simulink model "Position_Sliding_Mode"  (R2024b)
settings: Solver=ode4  StartTime=0.0  StopTime=20  FixedStep=dT  RelTol=1e-3
InitFcn:
  | O = [0; 0; 0];        % world origin frame
  | C = [0.0; 0.0; 0.0];  % camera origin frame
  | 
  | d_initial = C - O;            % distance between camera and world frame
  | ang_initial = [0.0 0.0 0.0];  % initial orientation, [pi 0 pi/2]
  | ang_final = [0.0*pi/180  0.0*pi/180  0.0*pi/180];
  | init_pose = [C ; ang_initial'];
  | d_final=[0; 0; 3];
  | dT=0.25;
  | g = 9.81;
  | mass = 1; L = 0.2;
  | Ix = 0.008;
  | Iy = 0.015;
  | Iz = 0.017;
  | c = 0.088;
settings Model: Creator=k513  LastModifiedBy=mohsen
settings ModelReferenceCC: EnableRefExpFcnMdlSchedulingChecks=on
settings RTWCC: GPUComputeCapability=3.5

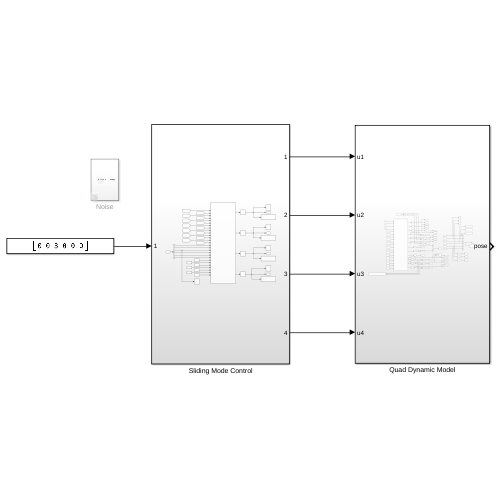
[thumbnail: Simulink's stored preview of the top-level diagram]
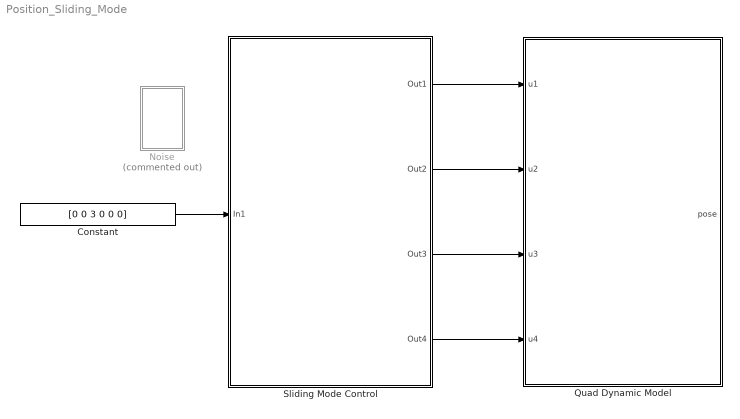
== system Position_Sliding_Mode ==
  Constant : Constant  Value=[0 0 3 0 0 0]
  Noise : Subsystem  Commented=on
  Quad Dynamic Model : Subsystem
  Sliding Mode Control : Subsystem
  wires:
  Sliding Mode Control/1(Out1) -> Quad Dynamic Model/1(u1)
  Sliding Mode Control/3(Out3) -> Quad Dynamic Model/3(u3)
  Sliding Mode Control/2(Out2) -> Quad Dynamic Model/2(u2)
  Sliding Mode Control/4(Out4) -> Quad Dynamic Model/4(u4)
  Constant/1 -> Sliding Mode Control/1(In1)

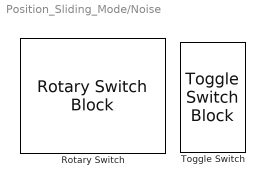
== system Position_Sliding_Mode/Noise ==
  Rotary Switch : RotarySwitchBlock  LabelPosition=Bottom
      settings: Values={{'Off', 'Low', 'Medium', 'High'}, [0 0.1 0.2 0.3]}
  Toggle Switch : ToggleSwitchBlock  LabelPosition=Bottom
      settings: Values={{'Off', 'On'}, [0 1]}

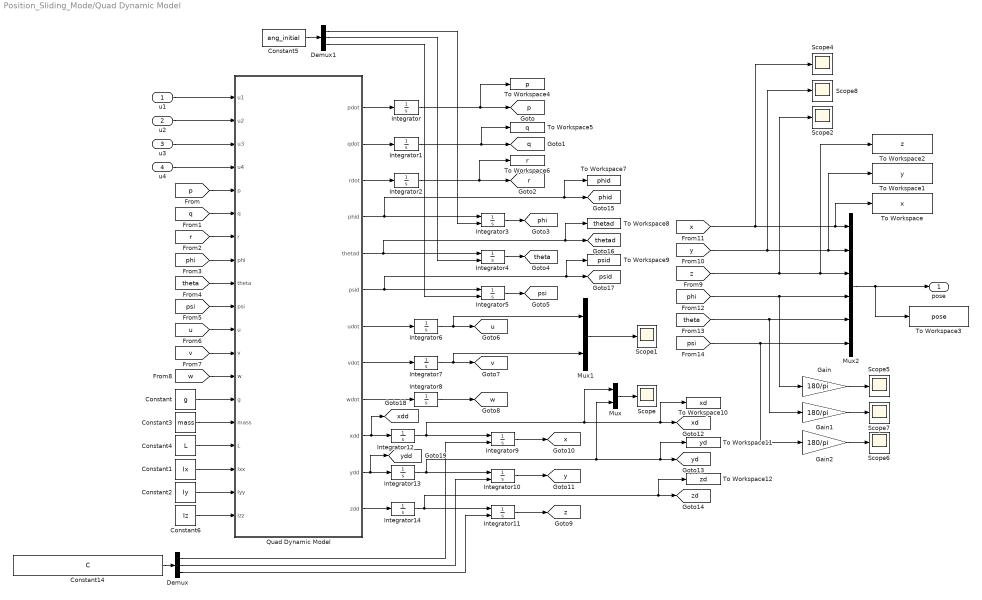
== system Position_Sliding_Mode/Quad Dynamic Model ==
  u1 : Inport
  u2 : Inport  Port=2
  u3 : Inport  Port=3
  u4 : Inport  Port=4
  Constant : Constant  Value=g
  Constant1 : Constant  Value=Ix
  Constant14 : Constant  Value=C
  Constant2 : Constant  Value=Iy
  Constant3 : Constant  Value=mass
  Constant4 : Constant  Value=L
  Constant5 : Constant  Value=ang_initial
  Constant6 : Constant  Value=Iz
  Demux : Demux  Outputs=3
  Demux1 : Demux  Outputs=3
  Gain : Gain  Gain=180/pi
  Gain1 : Gain  Gain=180/pi
  Gain2 : Gain  Gain=180/pi
  Integrator : Integrator  InitialCondition=-0.003775510005653
  Integrator1 : Integrator  InitialCondition=0.003931066952646
  Integrator{3..5,9..11} (6 alike) : Integrator  InitialConditionSource=external
  Integrator{6..8,12..14} (6 alike) : Integrator
  Integrator2 : Integrator  InitialCondition=0.005723309703171
  Mux : Mux  Inputs=2
  Mux1 : Mux  Inputs=2
  Mux2 : Mux  Inputs=6
  Quad Dynamic Model : MATLAB Function  TreatAsAtomicUnit=on
  Scope{,1..2,4..8} (8 alike) : Scope
  To Workspace : ToWorkspace  VariableName=x  SampleTime=-1
      settings: Save2DSignal=2-D array (concatenate along first dimension)
  To Workspace1 : ToWorkspace  VariableName=y  SampleTime=-1
      settings: Save2DSignal=2-D array (concatenate along first dimension)
  To Workspace10 : ToWorkspace  VariableName=xd  SampleTime=-1
  To Workspace11 : ToWorkspace  VariableName=yd  SampleTime=-1
  To Workspace12 : ToWorkspace  VariableName=zd  SampleTime=-1
  To Workspace2 : ToWorkspace  VariableName=z  SampleTime=-1
      settings: Save2DSignal=2-D array (concatenate along first dimension)
  To Workspace3 : ToWorkspace  VariableName=pose  SampleTime=-1
      settings: Save2DSignal=2-D array (concatenate along first dimension)
  To Workspace4 : ToWorkspace  VariableName=p  SampleTime=-1
  To Workspace5 : ToWorkspace  VariableName=q  SampleTime=-1
  To Workspace6 : ToWorkspace  VariableName=r  SampleTime=-1
  To Workspace7 : ToWorkspace  VariableName=phid  SampleTime=-1
  To Workspace8 : ToWorkspace  VariableName=thetad  SampleTime=-1
  To Workspace9 : ToWorkspace  VariableName=psid  SampleTime=-1
  pose : Outport
  tag scope: p=global, phi=global, phid=global, psi=global, psid=global, q=global, r=global, theta=global, thetad=global, u=global, v=global, w=global, x=global, xd=global, xdd=global, y=global, yd=global, ydd=global, z=global, zd=global
  wires:
  Quad Dynamic Model/1(pdot) -> Integrator/1
  Quad Dynamic Model/2(qdot) -> Integrator1/1
  Quad Dynamic Model/3(rdot) -> Integrator2/1
  Quad Dynamic Model/4(phid) -> To Workspace7/1, [phid], Integrator3/1
  Quad Dynamic Model/5(thetad) -> To Workspace8/1, [thetad], Integrator4/1
  Quad Dynamic Model/7(udot) -> Integrator6/1
  Quad Dynamic Model/9(wdot) -> Integrator8/1
  Quad Dynamic Model/10(xdd) -> [xdd], Integrator12/1
  Quad Dynamic Model/11(ydd) -> [ydd], Integrator13/1
  Quad Dynamic Model/12(zdd) -> Integrator14/1
  Integrator1/1 -> To Workspace5/1, [q]
  Integrator2/1 -> To Workspace6/1, [r]
  Integrator3/1 -> [phi]
  Integrator4/1 -> [theta]
  Integrator5/1 -> [psi]
  Integrator6/1 -> [u], Mux1/1
  Integrator7/1 -> [v], Mux1/2
  Integrator8/1 -> [w]
  [p] -> Quad Dynamic Model/5(p)
  [q] -> Quad Dynamic Model/6(q)
  [r] -> Quad Dynamic Model/7(r)
  [phi] -> Quad Dynamic Model/8(phi)
  [theta] -> Quad Dynamic Model/9(theta)
  [psi] -> Quad Dynamic Model/10(psi)
  [u] -> Quad Dynamic Model/11(u)
  [v] -> Quad Dynamic Model/12(v)
  [w] -> Quad Dynamic Model/13(w)
  Integrator9/1 -> [x]
  Integrator10/1 -> [y]
  Integrator11/1 -> [z]
  u1/1 -> Quad Dynamic Model/1(u1)
  u2/1 -> Quad Dynamic Model/2(u2)
  u3/1 -> Quad Dynamic Model/3(u3)
  u4/1 -> Quad Dynamic Model/4(u4)
  Integrator12/1 -> Mux/1, To Workspace10/1, [xd], Integrator9/1
  Integrator13/1 -> Mux/2, To Workspace11/1, [yd], Integrator10/1
  Integrator14/1 -> To Workspace12/1, [zd], Integrator11/1
  Quad Dynamic Model/6(psid) -> Integrator5/1, To Workspace9/1, [psid]
  Demux/1 -> Integrator9/2
  Demux/2 -> Integrator10/2
  Demux/3 -> Integrator11/2
  Mux/1 -> Scope/1
  Mux1/1 -> Scope1/1
  Constant14/1 -> Demux/1
  Quad Dynamic Model/8(vdot) -> Integrator7/1
  [x] -> Mux2/1, To Workspace/1, Scope4/1
  [phi] -> Gain/1, Mux2/4
  [psi] -> Mux2/6, Gain2/1
  [theta] -> Gain1/1, Mux2/5
  Gain/1 -> Scope5/1
  Gain1/1 -> Scope7/1
  Gain2/1 -> Scope6/1
  [y] -> Mux2/2, To Workspace1/1, Scope8/1
  [z] -> To Workspace2/1, Mux2/3, Scope2/1
  Mux2/1 -> pose/1, To Workspace3/1
  Constant/1 -> Quad Dynamic Model/14(g)
  Constant2/1 -> Quad Dynamic Model/18(Iyy)
  Constant1/1 -> Quad Dynamic Model/17(Ixx)
  Constant3/1 -> Quad Dynamic Model/15(mass)
  Constant4/1 -> Quad Dynamic Model/16(L)
  Constant5/1 -> Demux1/1
  Demux1/1 -> Integrator3/2
  Demux1/2 -> Integrator4/2
  Demux1/3 -> Integrator5/2
  Constant6/1 -> Quad Dynamic Model/19(Izz)
  Integrator/1 -> To Workspace4/1, [p]

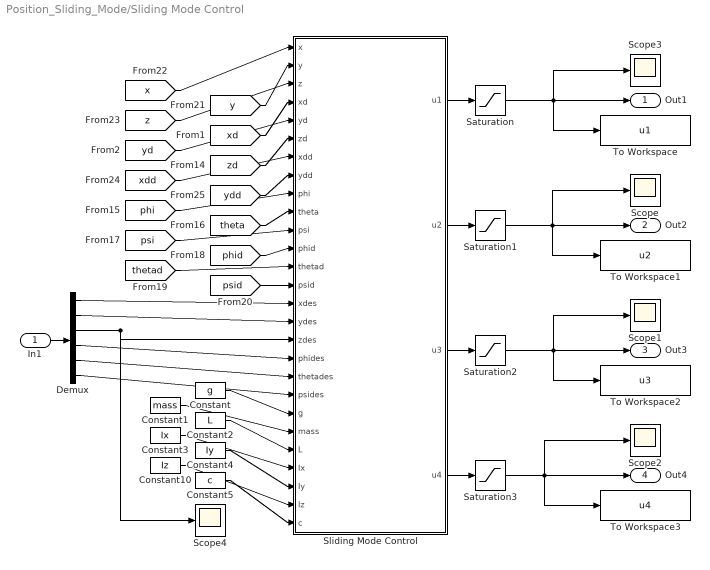
== system Position_Sliding_Mode/Sliding Mode Control ==
  In1 : Inport
  Constant : Constant  Value=g
  Constant1 : Constant  Value=mass
  Constant10 : Constant  Value=Iz
  Constant2 : Constant  Value=L
  Constant3 : Constant  Value=Ix
  Constant4 : Constant  Value=Iy
  Constant5 : Constant  Value=c
  Demux : Demux  Outputs=6
  Saturation : Saturate  UpperLimit=13  LowerLimit=9
  Saturation1 : Saturate  UpperLimit=8  LowerLimit=-8
  Saturation2 : Saturate  UpperLimit=8  LowerLimit=-8
  Saturation3 : Saturate  UpperLimit=4  LowerLimit=-3
  Scope{,1..4} (5 alike) : Scope
  Sliding Mode Control : MATLAB Function  TreatAsAtomicUnit=on
  To Workspace : ToWorkspace  VariableName=u1  SaveFormat=Timeseries  SampleTime=-1
  To Workspace1 : ToWorkspace  VariableName=u2  SaveFormat=Timeseries  SampleTime=-1
  To Workspace2 : ToWorkspace  VariableName=u3  SaveFormat=Timeseries  SampleTime=-1
  To Workspace3 : ToWorkspace  VariableName=u4  SaveFormat=Timeseries  SampleTime=-1
  Out1 : Outport
  Out2 : Outport  Port=2
  Out3 : Outport  Port=3
  Out4 : Outport  Port=4
  wires:
  [theta] -> Sliding Mode Control/10(theta)
  [zd] -> Sliding Mode Control/6(zd)
  [yd] -> Sliding Mode Control/5(yd)
  Sliding Mode Control/1(u1) -> Saturation/1
  [xdd] -> Sliding Mode Control/7(xdd)
  [thetad] -> Sliding Mode Control/13(thetad)
  [phid] -> Sliding Mode Control/12(phid)
  [psi] -> Sliding Mode Control/11(psi)
  Saturation/1 -> To Workspace/1, Out1/1, Scope3/1
  [ydd] -> Sliding Mode Control/8(ydd)
  [y] -> Sliding Mode Control/2(y)
  [phi] -> Sliding Mode Control/9(phi)
  [xd] -> Sliding Mode Control/4(xd)
  Sliding Mode Control/4(u4) -> Saturation3/1
  Sliding Mode Control/2(u2) -> Saturation1/1
  [psid] -> Sliding Mode Control/14(psid)
  [x] -> Sliding Mode Control/1(x)
  [z] -> Sliding Mode Control/3(z)
  Sliding Mode Control/3(u3) -> Saturation2/1
  Saturation2/1 -> To Workspace2/1, Out3/1, Scope1/1
  Saturation1/1 -> To Workspace1/1, Out2/1, Scope/1
  Saturation3/1 -> Scope2/1, To Workspace3/1, Out4/1
  In1/1 -> Demux/1
  Demux/1 -> Sliding Mode Control/15(xdes)
  Demux/2 -> Sliding Mode Control/16(ydes)
  Demux/3 -> Scope4/1, Sliding Mode Control/17(zdes)
  Constant/1 -> Sliding Mode Control/21(g)
  Constant1/1 -> Sliding Mode Control/22(mass)
  Constant2/1 -> Sliding Mode Control/23(L)
  Constant3/1 -> Sliding Mode Control/24(Ix)
  Constant4/1 -> Sliding Mode Control/25(Iy)
  Constant5/1 -> Sliding Mode Control/27(c)
  Demux/5 -> Sliding Mode Control/19(thetades)
  Demux/6 -> Sliding Mode Control/20(psides)
  Demux/4 -> Sliding Mode Control/18(phides)
  Constant10/1 -> Sliding Mode Control/26(Iz)

== matlab function Position_Sliding_Mode/Quad Dynamic Model/Quad Dynamic Model ==
  data: u1 input; u2 input; u3 input; u4 input; p input; pdot output; q input; r input; qdot output; rdot output; phi input; theta input; psi input; u input; v input; w input; phid output; thetad output; psid output; udot output; vdot output; wdot output; xdd output; ydd output; zdd output; g input; mass input; L input; Ixx input; Iyy input; Izz input
function [pdot, qdot, rdot, phid, thetad, psid, udot, vdot, wdot, xdd, ydd, zdd] = fcn(u1, u2, u3, u4, p, q, r, phi, theta, psi, u, v, w, g, mass, L, Ixx, Iyy, Izz)


% k1 = 0.1; k2 = 0.1; k3 = 0.1; k4 = 0.12; k5 = 0.12; k6 = 0.12;
%Izz = Ixx+Iyy;

pdot = r*q*(Iyy - Izz)/Ixx + L*(u2)/Ixx;
qdot = r*p*(Izz - Ixx)/Iyy + L*(u3)/Iyy;
rdot = p*q*(Ixx - Iyy)/Izz + L*(u4)/Izz;

phid = p + q*sin(phi)*tan(theta) + r*cos(phi)*tan(theta);
thetad = q*cos(phi) - r*sin(phi);
psid = q*sin(phi)*sec(theta) + r*cos(phi)*sec(theta);

udot = r*v - q*w -g*sin(theta);
vdot = p*w - u*r +g*cos(theta)*sin(phi); 
wdot = q*u - p*v +g*cos(theta)*cos(phi) - u1/mass;

% AA = [cos(psi)*cos(theta), -sin(psi)*cos(phi)+cos(psi)*sin(theta)*sin(phi), sin(psi)*sin(phi)+cos(psi)*sin(theta)*cos(phi);
%      sin(psi)*cos(theta), cos(psi)*cos(phi)+sin(psi)*sin(theta)*sin(phi), -sin(phi)*cos(psi)+sin(psi)*sin(theta)*cos(phi);
%     -sin(theta), cos(theta)*sin(phi), cos(theta)*cos(phi)]; 
% 
% xd = AA(1,:)*[u;v;w];
% yd = AA(2,:)*[u;v;w];
% zd = AA(3,:)*[u;v;w];

% xdd = (-u1/mass)*(sin(phi)*sin(psi)+cos(phi)*cos(psi)*sin(theta));
% ydd = (-u1/mass)*(cos(phi)*sin(psi)*sin(theta)-cos(psi)*sin(phi));
% zdd = g + (-u1/mass)*(cos(phi)*cos(theta));

xdd = (1/mass)*(cos(phi)*sin(theta)*cos(psi)+sin(phi)*sin(psi))*u1;
ydd = (1/mass)*(sin(psi)*sin(theta)*cos(phi)-cos(psi)*sin(phi))*u1;
zdd = -(1/mass)*(cos(phi)*cos(theta))*u1+g;

== matlab function Position_Sliding_Mode/Sliding Mode Control/Sliding Mode Control ==
  data: u1 output; x input; y input; z input; xd input; yd input; zd input; xdd input; ydd input; phi input; theta input; psi input; phid input; thetad input; psid input; xdes input; ydes input; zdes input; phides input; thetades input; u2 output; u3 output; u4 output; psides input; g input; mass input; L input; Ix input; Iy input; Iz input; c input
function [u1, u2, u3, u4] = fcn(x,y,z,xd,yd,zd,xdd,ydd,phi,theta,psi,phid,thetad,psid, xdes, ydes, zdes,phides, thetades,psides,g,mass,L,Ix,Iy,Iz, c)

%g = 9.81;
%mass = 1; L = 0.6; 
%Ix = 0.85; 
%Iy = 0.85; 
%Iz = Ix+Iy;
%c = 0.088; 
phiddes = 0;
phidddes = 0;

%thetades = 0.0*pi/180;
thetaddes = 0;
thetadddes = 0;
%phides = 0.0*pi/180;

%xdes = 0;
xddes = 0;
xdddes = 0;
%ydes = 0;
yddes = 0;
ydddes = 0;
% zdes = 0;
zddes = 0;
zdddes = 0;
% psides = 0*pi/180;
psiddes = 0;
psidddes = 0;

%phides=0;
%thetades=0;
%if zdes<0
%    zdes=0.5;
%end

%%
ghat = 1 * g; cz = 1; masshat = mass;
eps1 = 0.8;
eta1 = 1;
s1 = cz*(z - zdes) + (zd - zddes);
% if s1 > 1
%     sgn1 = 1;
% elseif   s1 < -1
%     sgn1 = -1;
% else
%     sgn1 = s1;
% end
sgn1 = tanh(s1);
u1 = (masshat/(cos(phi)*cos(theta)))*(cz*(zd-(zddes)) + zdddes + ghat + eps1*sgn1 + eta1*s1);
%%
cpsi = 1.5; eps2 = .8; eta2 = 2; 
Izhat = 1 * Iz; chat = 1 * c;
s2 = cpsi*(psides - psi) + (psiddes - psid);
% if s2 > 1
%     sgn2 = 1;
% elseif   s2 < -1
%     sgn2 = -1;
% else
%     sgn2 = s2;
% end
sgn2 = tanh(s2);
u4 = (Izhat/chat)*(cpsi*(psiddes-psid) + psidddes + eps2*sgn2 + eta2*s2);
%% 
eps3 = 0.5; eta3 = 5; ctheta = 1.5;
Iyhat = 1 * Iy; Ixhat = 1 * Ix; lhat = 1 * L;
c3 = 1;
% c1 = (11*mass/(u1*cos(phi)*cos(psi)*cos(thetades))) * c3;
% c2 = (6*mass/(u1*cos(phi)*cos(psi)*cos(thetades))) * c3;
c1 = (11*mass/(cos(phi)*cos(psi)*cos(thetades))) * c3;
c2 = (6*mass/(cos(phi)*cos(psi)*cos(thetades))) * c3;
c4 = (6) * c3;
s3 = c1*(xddes - xd) + c2*(xdes - x) + c3*(thetaddes - thetad) + c4*(thetades - theta);
% s3 = c3*(thetaddes - thetad) + c4*(thetades- theta);

% if s3 > 1
%     sgn3 = 1;
% elseif   s3 < -1
%     sgn3 = -1;
% else
%     sgn3 = s3;
% end
sgn3 = tanh(s3);
u3 = (Iyhat/lhat)*((c1/c3)*(xdddes-xdd) + (c2/c3)*(xddes-xd) + thetadddes ...
       + (c4/c3)*(thetaddes-thetad)  + (1/c3)*(eps3*sgn3 + eta3*s3));

% u3 = (Iyhat/chat)*(ctheta*(thetaddes-thetad) + thetadddes + eps3*sgn3 + eta3*s3);

%u3(st) = 0;
%%
eps4 = 0.5; eta4 = 5; chphi = 1.5;
c7 = 1;
% c5 = (-11*mass/((u1*sin(phides)*sin(theta)*sin(psi))+(u1*cos(phides)*cos(psi)))) * c7;
% c6 = (-6*mass/((u1*sin(phides)*sin(theta)*sin(psi))+(u1*cos(phides)*cos(psi)))) * c7;
% c5 = (-11*mass/((sin(phides)*sin(theta)*sin(psi))+(u1*cos(phides)*cos(psi)))) * c7;
% c6 = (-6*mass/((sin(phides)*sin(theta)*sin(psi))+(u1*cos(phides)*cos(psi)))) * c7;
c5 = (-11*mass/((sin(phides)*sin(theta)*sin(psi))+(cos(phides)*cos(psi)))) * c7;
c6 = (-6*mass/((sin(phides)*sin(theta)*sin(psi))+(cos(phides)*cos(psi)))) * c7;
c8 = (6) * c7;
s4 = c5*(yddes - yd) + c6*(ydes - y) + c7*(phiddes - phid) + c8*(phides - phi);
% s4 = c7*(phiddes - phid) + c8*(phides - phi);
% if s4 > 1
%     sgn4 = 1;
% elseif   s4 < -1
%     sgn4 = -1;
% else
%     sgn4 = s4;
% end
sgn4 = tanh(s4);
u2 = (Ixhat/lhat)*((c5/c7)*(ydddes-ydd) + (c6/c7)*(yddes-yd) + phidddes ...
        + (c8/c7)*(phiddes-phid) +  (1/c7)*(eps4*sgn4 + eta4*s4));
% u2 = (Ixhat/lhat)*(chphi*(phiddes-phid) + phidddes + eps4*sgn4 + eta4*s4);
